simulink model "acc_with_sensor_copy"  (R2021b)
settings: Solver=FixedStepAuto  StartTime=0.0  StopTime=206  FixedStep=0.0005  RelTol=1e-3
InitFcn:
  | G=9.81;
  | m=1660;
  | rw=0.325;
  | Caf=74070;
  | Car=58525;
  | Iz=2778.5;
  | d = 1.502;
  | lf =1.1135;
  | lr =1.5065;
  | L = 2.62;
  | kph2mps=1/3.6;
values from neighbouring files (symbols this model uses):
  Leftdis_PV_switch = 2    [acc_plot_backup.m]
  s_path = [0 1.10508939428 2.2141958029 3.32141571172 4.42705301151 5.53154548532 6.63517443471 7.73808041313 8.84055018688 9.94289959674 11.0453539299 12.1480581097 ... (1001 elements, 1001x1)]    [200_100radius.mat]    (also in LV_Clothoid_S_Turn_path.mat = [0 0.966832089581 1.93621320584 2.90214024471 3.86476766313 ; NEDC_path.mat = [0 0.414605943146 0.832514087334 1.25401518562 1.68216660344; Straight_East_into_curve.mat = [0 1.65770560069 3.32192925577 4.98420060507 6.64484613518 8; acc_plot_backup.m = Station_HV_m)
  X_path = [0 1.10508939428 2.2141958029 3.32141571172 4.42705301151 5.53154548532 6.63517443471 7.73808041313 8.84055018688 9.94289959674 11.0453539299 12.1480581097 ... (1001 elements, 1001x1)]    [200_100radius.mat]    (also in LV_Clothoid_S_Turn_path.mat = [-10 -9.03316791042 -8.06378679416 -7.09785975529 -6.1352323; NEDC_path.mat = [0 0.414605943146 0.832514087334 1.25401518562 1.68216660344; Straight_East_into_curve.mat = [0 1.65770560069 3.32192925577 4.98420060507 6.64484613518 8; acc_plot_backup.m = X_HV_m)
  Y_path = [0 -1.70364610795e-18 -7.41532896709e-18 1.46822109542e-17 4.74557362791e-17 6.12980216762e-17 9.25043977736e-17 1.24088240159e-16 1.5099156923e-16 1.7058517853e-16 1.90629227614e-16 2.09673434424e-16 ... (1001 elements, 1001x1)]    [200_100radius.mat]    (also in LV_Clothoid_S_Turn_path.mat = [0 -8.46153035536e-19 5.07382551045e-18 2.07356032218e-17 3.; NEDC_path.mat = [0 -3.50680326162e-18 -2.14111304971e-18 3.38197671014e-18 3; Straight_East_into_curve.mat = [0 1.29197709199e-18 2.81882429322e-18 3.49020462564e-17 6.7; acc_plot_backup.m = Y_HV_m)
undefined symbols (not defined in the file or in its folder): C_TICK_TIME_S, Cut_in_Secenary_flg, ENUM_ACCSTATE_DISABLED, ENUM_ACCSTATE_OFF, ENUM_ACCSTATE_STANDBY, FALSE, KVDI_ACCLongPressTime_ms, KVDI_ACCMaxActSpeed_kph, KVDI_ACCSetSpdIntial_kph, KVDI_ACCSpdLargeChange_kph, KVDI_LongPressConTime_ms, ONE_FLOAT, ONE_INT, Path_selector, R, Rw, T, TRUE, UseTTC_switch, ZERO_FLOAT, ZERO_INT
libraries: simulink x15, dspstat3 x4, simulink_extras x2, Solver_SF x1
(part 1 of 8)
settings Model: Creator=power  LastModifiedBy=power
settings DataIOCC: ReturnWorkspaceOutputs=off

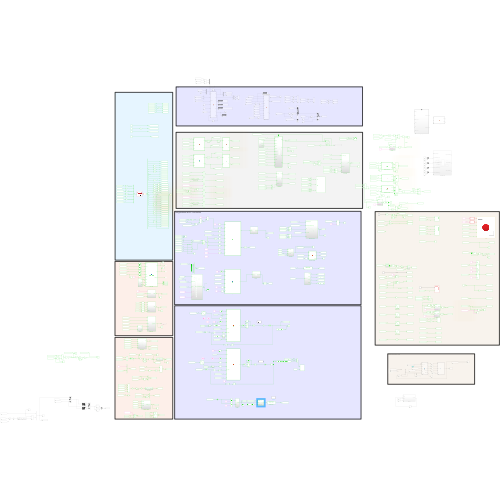
[thumbnail: Simulink's stored preview of the top-level diagram]
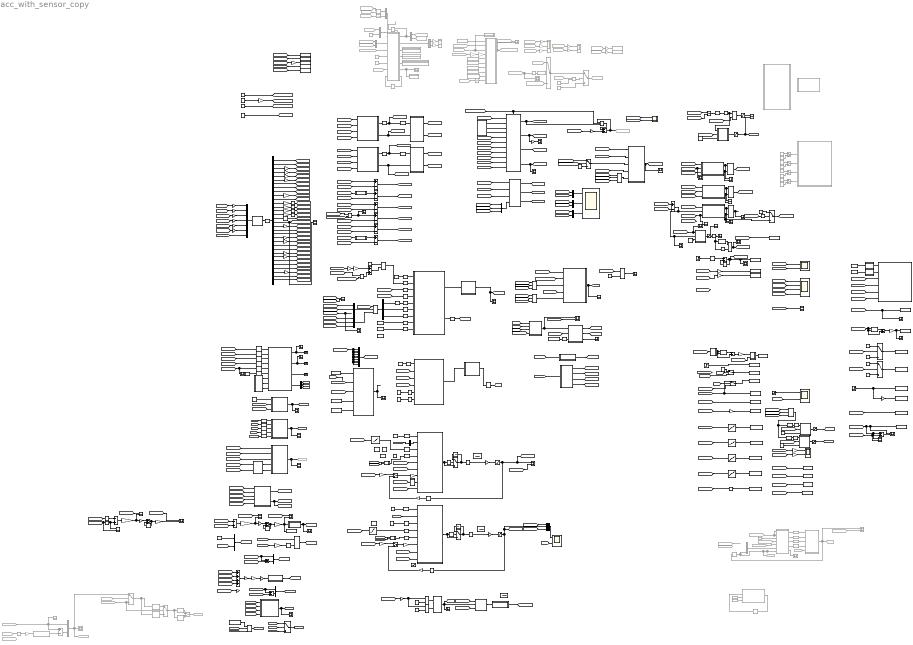
== system acc_with_sensor_copy ==
  note: Lateral MPC controller
  note: Kalman Filter
  note: Carsim
  note: Record data
  note: Longitudinal MPC controller
  note: Camera_emulator
  note: Longitudinal Constraint MPC controller
  note: Doesn't work with low speed
  note: Estimator
  note: Car_following_trajectory_planning
  1-D Lookup Table Accel Limit1 : Lookup_n-D  NumberOfTableDimensions=1  BreakpointsForDimension1=[0,5,20,30]  Table=[4,4,2,2]  InternalRulePriority=Speed  RndMeth=Simplest  InputSameDT=on
  1-D Lookup Table Deccel Limit2 : Lookup_n-D  NumberOfTableDimensions=1  BreakpointsForDimension1=[0,5,20,30]  Table=[-5,-5,-2.5,-2.5]  InternalRulePriority=Speed  RndMeth=Simplest  InputSameDT=on
  1-D Lookup Table Jerk LowLimit1 : Lookup_n-D  NumberOfTableDimensions=1  BreakpointsForDimension1=[0,5,20,30]  Table=[-5,-5,-2.5,-2.5]  InternalRulePriority=Speed  RndMeth=Simplest  InputSameDT=on
  1-D Lookup Table Jerk UpLimit1 : Lookup_n-D  NumberOfTableDimensions=1  BreakpointsForDimension1=[0,5,20,30]  Table=[5,5,2.5,2.5]  InternalRulePriority=Speed  RndMeth=Simplest  InputSameDT=on
  1-D Lookup Table1 : Lookup_n-D  NumberOfTableDimensions=1  BreakpointsForDimension1=[35 40 70 80]/3.6  Table=[0.01 0.01 0.0025 0.0025]  InternalRulePriority=Speed  RndMeth=Simplest  InputSameDT=on
  1-D Lookup Table2 : Lookup_n-D  NumberOfTableDimensions=1  BreakpointsForDimension1=[0 10 35 40]/3.6  Table=[0.25 0.25 0.025 0.025]  InternalRulePriority=Speed  RndMeth=Simplest  InputSameDT=on
  11:20 : Selector  Commented=on  InputPortWidth=20  IndexOptions=Index vector (dialog)  Indices=[11:20]  OutputSizes=1
  1:10 : Selector  Commented=on  InputPortWidth=20  IndexOptions=Index vector (dialog)  Indices=[1:10]  OutputSizes=1
  ACCSpdCalculation : Subsystem  Commented=on
  ACC_Mode_Selector : Subsystem
  Abs{,1..2,4} (4 alike) : Abs
  Abs6 : Abs  Commented=on
  Acceleration controller2 : MATLAB Function  TreatAsAtomicUnit=on
  Add{,1..3,13..14,16..17,20,32} (10 alike) : Sum  Inputs=+-
  Add Constant : Bias  Bias=-2
  Add Constant1 : Bias  Bias=2
  Add Constant2 : Bias  Bias=-2
  Add Constant4 : Bias  Bias=+2
  Add Constant5 : Bias  Bias=-2
  Add{4,9..10,60} (4 alike) : Sum  Inputs=-+
  Add{6,11,15,18,62} (5 alike) : Sum
  Add26 : Sum  Commented=on  Inputs=+-
  Add56 : Sum  Inputs=++++
  Camera_NEW : MATLAB Function  TreatAsAtomicUnit=on
  CarSim S-Function : Solver_SF/CarSim S-Function  Priority=1  SIMFILE=simfile.sim  Run_RTs=off  vs_state_ind=Run  StopMode_ind=Vehicle Model
  Compare To Constant2 : simulink/Logic and Bit Operations/Compare To Constant  Commented=on  relop=>  const=.015  OutDataTypeStr=boolean
  Compare To Constant4 : simulink/Logic and Bit Operations/Compare To Constant  relop===  const=0  OutDataTypeStr=boolean
  Compare To Constant5 : simulink/Logic and Bit Operations/Compare To Constant  relop=>=  const=2  OutDataTypeStr=boolean
  Constant : Constant  Value=0  SampleTime=0.1
  Constant10 : Constant  Value=0.1
  Constant11 : Constant  Value=45  SampleTime=0.1
  Constant111 : Constant  Value=10
  Constant{12..13,24,45} (4 alike) : Constant  Commented=on  OutDataTypeStr=boolean
  Constant14 : Constant  Value=1270+22*4+88.6+54.4  SampleTime=0.1
  Constant{15,39,46..47} (4 alike) : Constant  Commented=on  Value=0  OutDataTypeStr=boolean
  Constant{9,16,28,40,58,92} (6 alike) : Constant
  Constant17 : Constant  Value=0.3
  Constant18 : Constant  Value=0.025
  Constant19 : Constant  Value=0  SampleTime=0.1
  Constant2 : Constant  Value=2
  Constant20 : Constant  Value=10
  Constant21 : Constant  Value=10  SampleTime=0.1
  Constant{7,22,29,36,49,53} (6 alike) : Constant  Value=1.5
  Constant23 : Constant  Value=1.5  SampleTime=0.1
  Constant25 : Constant  Commented=on  Value=0.3
  Constant26 : Constant  Value=X_path
  Constant27 : Constant  Value=Y_path
  Constant3 : Constant  Value=0.1
  Constant30 : Constant  Value=35
  Constant31 : Constant  Value=3
  Constant32 : Constant  Value=30
  Constant33 : Constant  Value=5
  Constant34 : Constant  Value=-3
  Constant35 : Constant  Value=-5
  Constant37 : Constant  Commented=on  Value=0.1
  Constant38 : Constant  Commented=on  Value=0
  Constant4 : Constant  Value=0.0025
  Constant41 : Constant  Value=0.01
  Constant42 : Constant  Value=0.5
  Constant43 : Constant  Value=0.0125
  Constant44 : Constant  Commented=on  Value=100
  Constant48 : Constant  Commented=on  Value=75
  Constant5 : Constant  Value=0.2
  Constant50 : Constant  Commented=on  Value=3
  Constant52 : Constant  Commented=on  Value=1.015
  Constant54 : Constant  Commented=on  Value=2.910-1.015
  Constant55 : Constant  Commented=on  Value=1270+22*4+88.6+54.4
  Constant56 : Constant  Commented=on  Value=0.1
  Constant57 : Constant  Commented=on  Value=73922.12
  Constant59 : Constant  Commented=on  Value=54682
  Constant6 : Constant  Value=2.5
  Constant60 : Constant  Commented=on  Value=15/3.6
  Constant61 : Constant  Commented=on  Value=0
  Constant62 : Constant  Value=Leftdis_PV_switch
  Constant63 : Constant  Value=0
  Constant67 : Constant  SampleTime=0.1
  Constant8 : Constant  SampleTime=0.1
  Cos : Trigonometry  Operator=tan
  Cut-in strategy : Subsystem
  Delay{,3..4,7} (4 alike) : Delay  DelayLength=1  SampleTime=0.1
  Delay1 : Delay  DelayLength=1
  Delay10 : Delay  Commented=on  DelayLength=1  InitialConditionSource=Input port  InitialCondition=[50/3.6 0]'  SampleTime=0.1
      settings: InputPortMap=u0,p4
  Delay2 : Delay  DelayLength=1  InitialConditionSource=Input port  SampleTime=0.1
      settings: InputPortMap=u0,p4
  Delay48 : Delay  Commented=on  DelayLength=1  InitialCondition=[1 0;0 1]  SampleTime=0.1
  Delay49 : Delay  Commented=on  DelayLength=1  InitialConditionSource=Input port  InitialCondition=[50/3.6 0]'  SampleTime=0.1
      settings: InputPortMap=u0,p4
  Delay5 : Delay  Commented=on  DelayLength=1  SampleTime=0.1
  Delay50 : Delay  DelayLength=1
  Delay6 : Delay  DelayLength=1  InitialConditionSource=Input port  SampleTime=0.1
      settings: InputPortMap=u0,p4
  Delay8 : Delay  Commented=on  DelayLength=1  SampleTime=0.1
  Delay9 : Delay  DelayLength=1  InitialConditionSource=Input port  ExternalReset=Rising  SampleTime=0.1
      settings: InputPortMap=u0,r5,p4
  Demux : Demux  Outputs=32
  Demux14 : Demux
  Demux2 : Demux  Outputs=[10]
  Demux3 : Demux  Outputs=3
  Demux6 : Demux  Commented=on  Outputs=2
  Demux8 : Demux  Commented=on  Outputs=2
  Detect Increase : simulink/Logic and Bit Operations/Detect Increase  vinit=0.0  OutDataTypeStr=boolean
  Display{,4..7} (5 alike) : Display  Commented=on
      Display4 settings: Format=bank
      Display5 settings: Format=bank
      Display6 settings: Format=bank
      Display7 settings: Format=bank
  Divide : Product  Inputs=*/
  Divide1 : Product  Inputs=*/
  Estimation_TTCx_PV : MATLAB Function  TreatAsAtomicUnit=on
  Estimation_TTCx_PV1 : MATLAB Function  TreatAsAtomicUnit=on
  Estimation_TTCx_PV2 : MATLAB Function  TreatAsAtomicUnit=on
  Estimation_TTCy_PV : MATLAB Function  Commented=on  TreatAsAtomicUnit=on
  From149 : From  Commented=on  GotoTag=Ax_HV_mps2
  From157 : From  Commented=on  GotoTag=Vx_p
  From159 : From  Commented=on  GotoTag=ACCSetSpeed_mps
  From{80,160,237,247..248,253} (6 alike) : From  Commented=on  GotoTag=Vx_HV_mps
  From161 : From  Commented=on  GotoTag=Ax_HV_mps2
  From163 : From  Commented=on  GotoTag=RR
  From{166,180,232,238} (4 alike) : From  Commented=on  GotoTag=Vy_HV_mps
  From{167,219,234,258,273} (5 alike) : From  Commented=on  GotoTag=Vy_e_output
  From175 : From  Commented=on  GotoTag=Ry
  From188 : From  Commented=on  GotoTag=x_translate
  From193 : From  Commented=on  GotoTag=Ry
  From216 : From  Commented=on  GotoTag=Yaw_rate_radps
  From217 : From  Commented=on  GotoTag=Yaw_rate_radps
  From221 : From  Commented=on  GotoTag=Steer_SW_deg
  From233 : From  Commented=on  GotoTag=Ay_HV_mps2
  From239 : From  Commented=on  GotoTag=Estimated_Vx_mps
  From241 : From  Commented=on  GotoTag=Yaw_rate_radps
  From242 : From  Commented=on  GotoTag=Vy_e_Small_YawRate
  From243 : From  Commented=on  GotoTag=Ax_HV_mps2
  From244 : From  Commented=on  GotoTag=Vy_e_Small_YawRate
  From245 : From  Commented=on  GotoTag=ax_c_old
  From246 : From  Commented=on  GotoTag=Ay_HV_mps2
  From255 : From  Commented=on  GotoTag=Estimated_Vy_mps
  From257 : From  Commented=on  GotoTag=Estimated_Vy_mps
  Gain : Gain  Gain=0.25
  Gain{1,9..10,15,47..49,58} (8 alike) : Gain  Gain=1/3.6
  Gain{11,17,45,56} (4 alike) : Gain  Gain=0.1
  Gain12 : Gain  Gain=0.5
  Gain{6,8,13,19..21,31..32} (8 alike) : Gain  Gain=3.6
  Gain{14,27,30,42} (4 alike) : Gain  Gain=pi/180
  Gain18 : Gain  Gain=[0:9]
  Gain22 : Gain  Gain=0.5
  Gain23 : Gain  Gain=20
  Gain{24..26,34} (4 alike) : Gain  Gain=1/20
  Gain28 : Gain  Gain=20
  Gain3 : Gain  Gain=9.81
  Gain{33,36..38} (4 alike) : Gain
  Gain35 : Gain  Gain=-1
  Gain4 : Gain  Gain=9.81
  Gain{40,43,51..55,80..81} (9 alike) : Gain  Commented=on  Gain=3.6
  Gain41 : Gain  Commented=on  Gain=1/20
  Gain44 : Gain  Commented=on  Gain=pi/180
  Gain46 : Gain  Commented=on  Gain=0.1
  Gain5 : Gain  Gain=180/pi
  Gain50 : Gain  Gain=9.81
  Gain{57,59..61} (4 alike) : Gain  Gain=pi/30
  Gain72 : Gain  Gain=180/pi
  Goto31 : Goto  Commented=on  GotoTag=ax_c_old
  Goto44 : Goto  Commented=on  GotoTag=spd_acc
  Goto49 : Goto  Commented=on  GotoTag=Estimated_Vx_mps
  Goto58 : Goto  Commented=on  GotoTag=RR
  Goto84 : Goto  Commented=on  GotoTag=Estimated_Vy_mps
  Goto90 : Goto  Commented=on  GotoTag=Vy_e_Small_YawRate
  Goto91 : Goto  Commented=on  GotoTag=Vy_e_output
  Goto93 : Goto  Commented=on  GotoTag=LeftDis_PV_multi
  Goto95 : Goto  Commented=on  GotoTag=y_translate
  IC : InitialCondition  Value=0
  Kalman_Filter_LatSpd1 : MATLAB Function  Commented=on  TreatAsAtomicUnit=on
  Latch : Subsystem
  LateralMotionKF1 : MATLAB Function  Commented=on  TreatAsAtomicUnit=on
  Logical Operator : Logic  Operator=NOT  AllPortsSameDT=off  OutDataTypeStr=boolean
  Logical Operator3 : Logic  AllPortsSameDT=off  OutDataTypeStr=boolean
  MATLAB Function1 : MATLAB Function  TreatAsAtomicUnit=on
  MATLAB Function10 : MATLAB Function  TreatAsAtomicUnit=on
  MATLAB Function13 : MATLAB Function  TreatAsAtomicUnit=on
  MATLAB Function17 : MATLAB Function  TreatAsAtomicUnit=on
  MATLAB Function3 : MATLAB Function  TreatAsAtomicUnit=on
  MATLAB Function4 : MATLAB Function  TreatAsAtomicUnit=on
  MATLAB Function5 : MATLAB Function  TreatAsAtomicUnit=on
  MATLAB Function6 : MATLAB Function  TreatAsAtomicUnit=on
  MPC : MATLAB Function  Commented=on  TreatAsAtomicUnit=on
  MPC_ACC : MATLAB Function  TreatAsAtomicUnit=on
  MPC_Bicycle_LDC1 : MATLAB Function  TreatAsAtomicUnit=on
  Manual Switch{,1,11..12} (4 alike) : ManualSwitch  Commented=on
  Manual Switch10 : ManualSwitch  Commented=on  CurrentSetting=0
  Manual Switch5 : ManualSwitch
  Manual Switch6 : ManualSwitch
  Manual Switch9 : ManualSwitch
  Min{,1..4} (5 alike) : MinMax  Inputs=2
  Multiport Switch{,1..4} (5 alike) : MultiPortSwitch  DataPortOrder=Zero-based contiguous  Inputs=2  DiagnosticForDefault=None  zeroidx=on
  Multiport Switch5 : MultiPortSwitch  Inputs=2
  Mux : Mux  Inputs=7
  Mux1 : Mux  Inputs=2
  Mux10 : Mux  Commented=on  Inputs=2
  Mux11 : Mux  Commented=on  Inputs=2
  Mux14 : Mux  Inputs=[1 19]
  Mux15 : Mux  Commented=on  Inputs=[1 19]
  Mux16 : Mux  Inputs=[1 19]
  Mux17 : Mux  Commented=on  Inputs=2
  Mux2 : Mux  Inputs=2
  Mux20 : Mux  Inputs=[1 19]
  Mux3 : Mux  Inputs=2
  Mux{4,6..8} (4 alike) : Mux  Inputs=3
  Mux5 : Mux  Inputs=10
  Mux9 : Mux  Commented=on  Inputs=[3 1 1 1]
  PV_trajectory_planning : Subsystem
  Product : Product
  Product2 : Product
  QP_logitudinal1 : MATLAB Function  Commented=on  TreatAsAtomicUnit=on
  Quantizer{1..6} (6 alike) : Quantizer  QuantizationInterval=0.02
  R selector : Subsystem
  R selector1 : Subsystem
  R1 : Constant  Value=0.5
  Radians to Degrees1 : simulink_extras/Transformations/Radians to Degrees
  Radians to Degrees2 : simulink_extras/Transformations/Radians to Degrees
  Rate Transition{1..5,18} (6 alike) : RateTransition  OutPortSampleTime=0.1
  Relational Operator : RelationalOperator  OutDataTypeStr=boolean  RndMeth=Simplest
  Relational Operator1 : RelationalOperator  Operator=<=  OutDataTypeStr=boolean  RndMeth=Simplest
  Relational Operator2 : RelationalOperator  Operator=isNaN  OutDataTypeStr=boolean  RndMeth=Simplest
  Relational Operator3 : RelationalOperator  Commented=on  OutDataTypeStr=boolean  RndMeth=Simplest
  Relational Operator4 : RelationalOperator  Operator=isNaN  OutDataTypeStr=boolean  RndMeth=Simplest
  Reshape : Reshape  Commented=on
  Saturation : Saturate  UpperLimit=100  LowerLimit=-100
  Saturation1 : Saturate  UpperLimit=10  LowerLimit=0
  Saturation2 : Saturate  UpperLimit=30/3.6  LowerLimit=5/3.6
  Saturation3 : Saturate  UpperLimit=720  LowerLimit=-720
  Saturation4 : Saturate  UpperLimit=400  LowerLimit=-400
  Saturation5 : Saturate  UpperLimit=2.5  LowerLimit=0
  Saturation6 : Saturate  UpperLimit=2.5  LowerLimit=0
  Saturation7 : Saturate  UpperLimit=10  LowerLimit=0
  Scope{,3..4,6..10,14..15,20,24,26,31..32,34,46,49,52,56,58..59,61,63..69,76,159} (32 alike) : Scope
  Scope{1..2,5,13,16..19,22,25,27,33,42..44,70..72,75} (19 alike) : Scope  NumInputPorts=2
  Scope11 : Scope  NumInputPorts=3
  Scope12 : Scope  NumInputPorts=4
  Scope21 : Scope  Commented=on  NumInputPorts=2
  Scope{23,30,36,38,41} (5 alike) : Scope  Commented=on
  Scope50 : Scope  Commented=on  NumInputPorts=2
  Smooth Switch : Subsystem
  Smooth Switch1 : Subsystem
  Smooth_Switch1 : Subsystem  mask{tau=0.3, IC=0, T=0.1}
      mask prompts: tau "Time constant"; T "Sample time"
      mask Display:
      | fprintf('Discrete first order \n\n')
      | fprintf(['tau=' num2str(tau) '    IC=' num2str(IC)])
  Smooth_Switch2 : Subsystem  mask{tau=0.3, IC=0, T=0.1}
      mask prompts: tau "Time constant"; T "Sample time"
      mask Display:
      | fprintf('Discrete first order \n\n')
      | fprintf(['tau=' num2str(tau) '    IC=' num2str(IC)])
  Step : Step  Time=0  Before=1.5  After=1.5  SampleTime=0
  Step1 : Step  Time=0  Before=1.5  After=1.5  SampleTime=0
  Step2 : Step  Time=0  After=0.1  SampleTime=0
  Step3 : Step  Time=0  Before=5  After=5  SampleTime=0.1
  Subsystem : Subsystem
  Subsystem1 : Subsystem
  Subsystem16 : Subsystem
  Subsystem17 : Subsystem
  Subsystem2 : Subsystem
  Subsystem3 : Subsystem
  Subsystem4 : Subsystem
  Subsystem5 : Subsystem
  Subsystem6 : Subsystem  Commented=on
  Subsystem7 : Subsystem
  Subsystem8 : Subsystem
  Switch : Switch  Criteria=u2 > Threshold
  Switch{1,8,11..13} (5 alike) : Switch  Criteria=u2 ~= 0
  Switch10 : Switch  Commented=on
  Switch2 : Switch  Commented=on  Criteria=u2 ~= 0
  Switch3 : Switch  Commented=on  Criteria=u2 > Threshold
  Switch4 : Switch  Criteria=u2 > Threshold
  Switch5 : Switch  Threshold=8
  Switch6 : Switch  Threshold=8
  Switch9 : Switch  Commented=on
  T : Gain  Gain=0.1
  T1 : Gain  Gain=0.1
  Terminator1 : Terminator
  Terminator2 : Terminator
  Terminator3 : Terminator
  To Workspace : ToWorkspace  VariableName=X_HV_m  SampleTime=-1
  To Workspace1 : ToWorkspace  VariableName=Y_HV_m  SampleTime=-1
  To Workspace10 : ToWorkspace  VariableName=TH  SampleTime=-1
  To Workspace11 : ToWorkspace  VariableName=RR  SampleTime=-1
  To Workspace12 : ToWorkspace  VariableName=Desired_distance  SampleTime=-1
  To Workspace13 : ToWorkspace  VariableName=C_tick_time  SampleTime=-1
  To Workspace14 : ToWorkspace  VariableName=Ax_HV_mps2  SampleTime=-1
  To Workspace15 : ToWorkspace  VariableName=V_ref_kph  SampleTime=-1
  To Workspace16 : ToWorkspace  VariableName=Ax_Up_Limit  SampleTime=-1
  To Workspace17 : ToWorkspace  VariableName=Ax_Low_Limit  SampleTime=-1
  To Workspace18 : ToWorkspace  VariableName=Jerk_x_Up_Limit  SampleTime=-1
  To Workspace19 : ToWorkspace  VariableName=Jerk_x_Low_Limit  SampleTime=-1
  To Workspace2 : ToWorkspace  VariableName=Yaw_HV_deg  SampleTime=-1
  To Workspace20 : ToWorkspace  VariableName=Acc_Mode  SampleTime=-1
  To Workspace21 : ToWorkspace  VariableName=Ay_Low_Limit  SampleTime=-1
  To Workspace22 : ToWorkspace  VariableName=Jerk_y_Up_Limit  SampleTime=-1
  To Workspace23 : ToWorkspace  VariableName=Jerk_y_Low_Limit  SampleTime=-1
  To Workspace24 : ToWorkspace  VariableName=Ay_HV_mps2  SampleTime=-1
  To Workspace25 : ToWorkspace  VariableName=y_error  SampleTime=-1
  To Workspace26 : ToWorkspace  VariableName=Steer_SW_deg  SampleTime=-1
  To Workspace29 : ToWorkspace  VariableName=TTC  SampleTime=-1
  To Workspace3 : ToWorkspace  VariableName=Station_HV_m  SampleTime=-1
  To Workspace30 : ToWorkspace  VariableName=X_APV_m  SampleTime=0.1
  To Workspace31 : ToWorkspace  VariableName=Y_APV_m  SampleTime=0.1
  To Workspace32 : ToWorkspace  VariableName=APV_kph  SampleTime=0.1
  To Workspace34 : ToWorkspace  VariableName=Ax_APV_mps2  SampleTime=0.1
  To Workspace36 : ToWorkspace  VariableName=Station_APV_m  SampleTime=0.1
  To Workspace4 : ToWorkspace  VariableName=Jerk_y  SampleTime=-1
  To Workspace40 : ToWorkspace  VariableName=Yaw_Est_deg  SampleTime=-1
  To Workspace42 : ToWorkspace  Commented=on  VariableName=Vy_HV_kph  SampleTime=-1
  To Workspace43 : ToWorkspace  Commented=on  VariableName=Vy_e_output  SampleTime=-1
  To Workspace5 : ToWorkspace  VariableName=Ay_Up_Limit  SampleTime=-1
  To Workspace6 : ToWorkspace  VariableName=HV_kph  SampleTime=-1
  To Workspace7 : ToWorkspace  VariableName=PV_kph  SampleTime=-1
  To Workspace8 : ToWorkspace  VariableName=Jerk_x  SampleTime=-1
  To Workspace9 : ToWorkspace  VariableName=TH_ref  SampleTime=0.1
  Transfer Fcn2 : TransferFcn  Denominator=[0.3 1]
  Transfer Fcn3 : TransferFcn  Denominator=[0.3 1]
  Transfer Fcn4 : TransferFcn  Denominator=[0.3 1]
  Unit Delay : UnitDelay  SampleTime=-1  HasFrameUpgradeWarning=on
  Unit Delay2 : UnitDelay  SampleTime=-1  HasFrameUpgradeWarning=on
  Unit Delay4 : UnitDelay  Commented=on  SampleTime=0.1  HasFrameUpgradeWarning=on
  Unit Delay5 : UnitDelay  Commented=on  SampleTime=0.1  HasFrameUpgradeWarning=on
  V_rel Estimation : Subsystem
  Vx4 : Scope  Commented=on  NumInputPorts=3
  Vx5 : Scope  Commented=on  NumInputPorts=2
  Vx6 : Scope  Commented=on  NumInputPorts=2
  XY Graph : Record  FileSettingsInternal="{\"entries\":[{\"content\":{\"excelSettings\":{\"content\":{},\"type\":\"Streamout.ExcelSettings\"}},\"type\":\"Streamout.FileSettingStorage\",\"uuid\":\"ae1c5602-517a-41a1-a61f-ee7d5eb1a325\"}],\"packageUris\":[\"http://schema.mathworks.com/mf0/streamout_blocks/R2020a\"],\"version\":\"1.0\"}"  Layout=[1 1]  SignalsInternal="{\"entries\":[{\"content\":{\"signals\":[{\"content\":{\"blockPath\":[\"acc_with_sensor/XY Graph\"],\"channel\":[],\"dimensions\":[1],\"domain\":\"acc_with_sensor/XY Graph\",\"lineColor\":\"#a2142f\",\"plots\":[1],\"port\":1,\"sid\":[\"\"],\"signalID\":8457,\"signalName\":\"x\"},\"type\":\"RecordBlkView.Signal\",\"uuid\":\"a7bf0323-9e6d-485d-a474-0a9d372fb7b1\"},{\"content\":{\"blockPath\":[\"acc_with_sensor/XY Graph\"],\"channel\":[],\"dimensions\":[1],\"domain\":\"acc_with_sensor/XY Graph\",\"lineColor\":\"#139fff\",\"plots\":[1],\"port\":2,\"sid\":[\"\"],\"signalID\":8461,\"signalName\":\"y\"},\"type\":\"RecordBlkView.Signal\",\"uuid\":\"749632c3-9221-4843-a7a6-8451e6d0203a\"},{\"content\":{\"blockPath\":[\"acc_with_sensor/XY Graph\"],\"channel\":[],\"dimensions\":[1],\"domain\":\"acc_with_sensor/XY Graph\",\"lineColor\":\"#64d413\",\"plots\":[1],\"port\":3,\"sid\":[\"\"],\"signalID\":8465,\"signalName\":\"X_HV\"},\"type\":\"RecordBlkView.Signal\",\"uuid\":\"02048bb8-c637-427d-932f-1a61c452e62e\"},{\"content\":{\"blockPath\":[\"acc_with_sensor/XY Graph\"],\"channel\":[],\"dimensions\":[1],\"domain\":\"acc_with_sensor/XY Graph\",\"lineColor\":\"#ff13a6\",\"plots\":[1],\"port\":4,\"sid\":[\"\"],\"signalID\":8469,\"signalName\":\"Y_HV\"},\"type\":\"RecordBlkView.Signal\",\"uuid\":\"63ffdeac-a074-4ec1-8896-dcf10e1ec4b5\"},{\"content\":{\"blockPath\":[\"acc_with_sensor/XY Graph\"],\"channel\":[],\"dimensions\":[1],\"domain\":\"acc_with_sensor/XY Graph\",\"lineColor\":\"#ff6929\",\"plots\":[1],\"port\":5,\"sid\":[\"\"],\"signalID\":8473,\"signalName\":\"X_PV\"},\"type\":\"RecordBlkView.Signal\",\"uuid\":\"92c1fdf2-3407-44d2-b4da-fad837cd08fa\"},{\"content\":{\"blockPath\":[\"acc_with_sensor/XY Graph\"],\"channel\":[],\"dimensions\":[1],\"domain\":\"acc_with_sensor/XY Graph\",\"lineColor\":\"#b746ff\",\"plots\":[1],\"port\":6,\"sid\":[\"\"],\"signalID\":8477,\"signalName\":\"Y_PV\"},\"type\":\"RecordBlkView.Signal\",\"uuid\":\"c8381700-cb77-42bf-bc65-a1a6c0c1696f\"}]},\"type\":\"RecordBlkView.InputSignals\",\"uuid\":\"40a95d25-711b-4f06-a3ff-602c17e43ef4\"}],\"packageUris\":[\"http://schema.mathworks.com/mf0/streamout_blocks/R2020a\"],\"version\":\"1.0\"}"  VisualizationBindings="{\"xyplotplugin\":{\"info\":[{\"series\":[{\"bindingParametersList\":[{\"parameter\":\"X-Axis\",\"signalID\":8465,\"signalName\":\"X_HV\"},{\"parameter\":\"Y-Axis\",\"signalID\":8469,\"signalName\":\"Y_HV\"}],\"seriesID\":54143},{\"bindingParametersList\":[{\"parameter\":\"X-Axis\",\"signalID\":8473,\"signalName\":\"X_PV\"},{\"parameter\":\"Y-Axis\",\"signalID\":8477,\"signalName\":\"Y_PV\"}],\"seriesID\":48964},{\"bindingParametersList\":[{\"parameter\":\"X-Axis\",\"signalID\":8457,\"signalName\":\"x\"},{\"parameter\":\"Y-Axis\",\"signalID\":8461,\"signalName\":\"y\"}],\"seriesID\":3520}],\"subplotID\":1}]}}"  CompatibilityTag=XY
  Zero-Order Hold{1..4,6,8..14,17..25,132..136} (26 alike) : ZeroOrderHold  SampleTime=0.1
  Zero-Order Hold{26..27,29,36} (4 alike) : ZeroOrderHold  Commented=on  SampleTime=0.1
  acceleration_apr1 : Subsystem
  acceleration_apr4 : Subsystem
  ascending : dspstat3/Sort  Commented=on  otype=Value  dir=Ascending  sortAlg=Quick sort  roundingMode=Floor  overflowMode=off  accumDataTypeStr=Inherit: Same as product output  accumLastDataTypeStr=Inherit: Same as product output
      settings: SourceProductBaseCode=DS
  car_length : Bias  Bias=-4.5
  car_length1 : Bias  Bias=4.5
  car_length2 : Bias  Bias=-4.5
  car_length3 : Bias  Bias=4.5
  cmd_limiter1 : Subsystem
  cmd_limiter4 : Subsystem
  descending : dspstat3/Sort  Commented=on  otype=Value  dir=Descending  sortAlg=Quick sort  roundingMode=Floor  overflowMode=off  accumDataTypeStr=Inherit: Same as product output  accumLastDataTypeStr=Inherit: Same as product output
      settings: SourceProductBaseCode=DS
  dist_safe : Bias  Bias=-2
  divide : Subsystem
  divide1 : Subsystem
  divide2 : Subsystem
  divide3 : Subsystem
  global to local2 : Subsystem
  global to local3 : Subsystem
  preview : Subsystem
  r/l : Gain  Gain=0.33415/1.675
  r/l1 : Gain  Gain=0.33415/1.675
  record_delta_x : Subsystem
  record_delta_yaw : Subsystem
  relative_dynamic_estimated : Subsystem  Commented=on
  rolling radius : Gain  Gain=0.325
  rolling_avg : Subsystem  Commented=on
  sample time1 : Gain  Gain=1/0.1
  sample time2 : Gain  Gain=1/0.1
  way2 : Goto  Commented=on  GotoTag=LeftDis_Camera
  tag scope: RAx_APV=global, RAx_PV=global, RR_APV=global, RR_PV=global, RVx_APV=global, RVx_PV=global, Vx_HV_mps=global
  wires:
  Demux/1 -> [X_HV_m]
  CarSim S-Function/1 -> Zero-Order Hold18/1
  Demux/2 -> [Y_HV_m]
  Demux/3 -> Gain9/1
  Demux/4 -> Gain10/1
  Demux/5 -> Gain3/1
  Demux/6 -> Gain4/1
  [Vx_PV_mps] -> Add1/1
  [Vx_HV_mps] -> Add1/2
  acceleration_apr4/1(acc_a) -> Add2/1  "PV"
  [Ax_HV_mps2] -> Add2/2  "HV"
  Constant14/1 -> Zero-Order Hold17/1
  Subsystem2/4(Pb_RR) -> [Braking_Pressure_RR]
  Product/1 -> Zero-Order Hold6/1
  [Driving_Brk_Cmd] -> Subsystem2/1(T_cmd)
  Subsystem2/1(Pb_LF) -> [Braking_Pressure_LF]
  Acceleration controller2/2(Tb) -> [Driving_Brk_Cmd]
  Acceleration controller2/3(Rtotal) -> Scope159/1
  Subsystem2/3(Pb_RL) -> [Braking_Pressure_RL]
  [Ax_HV_mps2] -> Zero-Order Hold9/1
  [Vx_HV_mps] -> Zero-Order Hold8/1
  Acceleration controller2/1(Tr) -> [Driving_Torque_Cmd]  "Torque"
  Subsystem2/2(Pb_RF) -> [Braking_Pressure_RF]
  Gain9/1 -> [Vx_HV_mps]
  Gain10/1 -> [Vy_HV_mps]
  Gain3/1 -> [Ax_HV_mps2]
  Gain4/1 -> [Ay_HV_mps2]
  Gain22/1 -> Mux/1  "Driving_Torque_FL"
  Gain12/1 -> Mux/2  "Driving_Torque_FR"
  Zero-Order Hold6/1 -> MATLAB Function1/2(Yref)
  Zero-Order Hold8/1 -> MATLAB Function1/3(Vx)
  Zero-Order Hold9/1 -> MATLAB Function1/4(ax)
  Zero-Order Hold10/1 -> MATLAB Function1/5(D_rel)
  Zero-Order Hold11/1 -> MATLAB Function1/6(V_rel)
  Zero-Order Hold12/1 -> MATLAB Function1/7(ax_rel)
  Zero-Order Hold13/1 -> MATLAB Function1/8(Qs)
  Zero-Order Hold14/1 -> MATLAB Function1/9(Rs)
  Abs/1 -> divide/1(dividend)
  Mux1/1 -> Scope11/1  "RR"
  [RR] -> Mux1/1  "RR"
  [RR_est] -> Mux1/2  "Est"
  [RVx] -> Mux2/1  "RV"
  [RV_est] -> Mux2/2  "Est"
  [RAx] -> Mux3/1  "RA"
  [RA_est] -> Mux3/2  "Est"
  Mux2/1 -> Scope11/2  "RV"
  Mux3/1 -> Scope11/3  "RA"
  [Braking_Pressure_RF] -> Gain36/1
  Gain33/1 -> Mux/3  "Driving_Torque_LF"
  [Braking_Pressure_LF] -> Gain33/1
  [Braking_Pressure_RL] -> Gain37/1
  Gain36/1 -> Mux/4  "Driving_Torque_RF"
  Gain38/1 -> Mux/6  "Driving_Torque_RR"
  Gain37/1 -> Mux/5  "Driving_Torque_RL"
  [Braking_Pressure_RR] -> Gain38/1
  [Braking_Pressure_LF] -> Scope12/1  "LF"
  [Braking_Pressure_RF] -> Scope12/2  "RF"
  [Braking_Pressure_RL] -> Scope12/3  "RL"
  [Braking_Pressure_RR] -> Scope12/4  "RR"
  MATLAB Function1/2(Y) -> Add Constant1/1  "MPC"
  Gain8/1 -> Scope18/1  "HV"
  Gain13/1 -> Scope18/2  "PV"
  [Vx_HV_mps] -> Acceleration controller2/2(Vxh)
  Zero-Order Hold17/1 -> Acceleration controller2/3(m)
  Zero-Order Hold18/1 -> Demux/1
  [RR] -> Scope13/2  "RR"
  Step/1 -> Scope2/1  "TH_limit"
  [TH] -> Scope2/2  "TH"
  Demux3/3 -> Zero-Order Hold12/1
  Zero-Order Hold3/1 -> MATLAB Function1/1(mode)
  [Driving_Torque] -> Gain22/1
  [Driving_Torque] -> Gain12/1
  [Ax_HV_mps2] -> Scope17/2  "ax_out"
  [Vx_HV_mps] -> Gain8/1  "HV"
  [Vx_PV_mps] -> Gain13/1  "PV"
  Demux3/2 -> Zero-Order Hold11/1
  [Driving_Torque_Cmd] -> Smooth_Switch2/1(In1)
  [Vx_HV_mps] -> MPC_ACC/3(Vx)
  [Ax_HV_mps2] -> MPC_ACC/4(ax)
  Constant92/1 -> Zero-Order Hold1/1
  Constant5/1 -> Zero-Order Hold2/1
  Constant2/1 -> Subsystem/4(Ax_max)
  Constant6/1 -> Subsystem/5(Jx_max)
  [Vx_HV_mps] -> Subsystem/3(VehSpd)
  [Vx_p] -> MPC_ACC/2(vx_p)
  Subsystem/1("VREF_LongiVehSpdRef_mps ") -> Scope4/1  "mps"
  Zero-Order Hold1/1 -> MPC_ACC/5(Qs)
  Zero-Order Hold2/1 -> MPC_ACC/6(Rs)
  MATLAB Function1/1(u) -> cmd_limiter1/1(ax_cmd)  "cmd"
  Add2/1 -> [RAx_PV]
  Add1/1 -> [RVx_PV]
  [Acc_Mode] -> ?
  [ACCSetSpeed_mps] -> Mux5/10, Mux5/9, Mux5/8, Mux5/7, Mux5/6, Mux5/5, Mux5/4, Mux5/3, Mux5/2, Mux5/1
  Add Constant/1 -> Abs/1
  Constant11/1 -> Gain15/1
  Gain15/1 -> [ACCSetSpeed_mps]
  Demux3/1 -> dist_safe/1
  [ACCSetSpeed_mps] -> ACC_Mode_Selector/1(ACCSetSpeed_mps)
  [VACCTargetVehAssigned_flg] -> ACC_Mode_Selector/2(VACCTargetVehNotAssigned_flg)
  [Vx_HV_mps] -> ACC_Mode_Selector/4(Vx_HV_mps)
  [Ax_HV_mps2] -> Gain17/1
  Gain17/1 -> Gain18/1
  Gain18/1 -> Add6/1
  Add6/1 -> Product/2  "Vp"
  Add Constant1/1 -> [Desired_distance]
  [Ax_PV_mps2] -> acceleration_apr4/1(acc_b)  "PV"
  Smooth_Switch2/1(Out1) -> [Driving_Torque]
  [Vx_HV_mps] -> Gain20/1  "HV"
  Gain19/1 -> To Workspace7/1  "PV"
  Gain20/1 -> To Workspace6/1  "HV"
  Subsystem4/1(new_ave) -> Delay2/1, Delay2/2, Add10/2
  Add10/1 -> sample time1/1
  Delay2/1 -> Add10/1
  sample time1/1 -> Subsystem3/1(Jerk)  "Jerk"
  Step1/1 -> To Workspace9/1  "TH_limit"
  [Desired_distance] -> Scope13/1  "Desired_distance"
  [Desired_distance] -> Switch8/1, To Workspace12/1  "Desired_distance"
  Step2/1 -> Delay3/1
  Add11/1 -> Scope31/1, To Workspace13/1, [C_tick_time], Delay/1
  Delay/1 -> Add11/2
  Delay3/1 -> Add11/1
  [Ax_HV_mps2] -> To Workspace14/1
  [ACCSetSpeed_mps] -> Subsystem/2(VehSpd_Ref)
  [ACCSetSpeed_mps] -> Gain21/1
  Gain21/1 -> To Workspace15/1
  Mux5/1 -> [Vx_p]
  Constant30/1 -> Relational Operator/2
  Relational Operator1/1 -> Latch/2(reset)
  Constant32/1 -> Relational Operator1/2
  Relational Operator/1 -> Latch/1(set)
  Gain31/1 -> Relational Operator/1, Relational Operator1/1  "kph"
  [RR_PV] -> Estimation_TTCx_PV/1(R)
  [RVx_PV] -> Estimation_TTCx_PV/2(V)
  [RAx_PV] -> Estimation_TTCx_PV/3(A)
  [Vx_HV_mps] -> 1-D Lookup Table Deccel Limit2/1
  1-D Lookup Table Deccel Limit2/1 -> To Workspace17/1
  [Vx_HV_mps] -> 1-D Lookup Table Accel Limit1/1
  1-D Lookup Table Accel Limit1/1 -> To Workspace16/1
  [Vx_HV_mps] -> 1-D Lookup Table Jerk UpLimit1/1
  [Vx_HV_mps] -> 1-D Lookup Table Jerk LowLimit1/1
  1-D Lookup Table Jerk UpLimit1/1 -> To Workspace18/1
  1-D Lookup Table Jerk LowLimit1/1 -> To Workspace19/1
  dist_safe/1 -> Zero-Order Hold10/1  "Drel"
  [Acc_Mode] -> Logical Operator/1
  Constant29/1 -> divide/3(default_value)
  divide/1(quotient) -> Saturation1/1
  Saturation1/1 -> [TH]  "TH_default"
  [X_PV_m] -> MATLAB Function3/1(Xf)
  [Y_PV_m] -> MATLAB Function3/2(Yf)
  [X_HV_m] -> MATLAB Function3/3(Xh)
  [Y_HV_m] -> MATLAB Function3/4(Yh)
  MATLAB Function3/1(RR) -> car_length/1  "RR_XY"
  Demux/7 -> [Station_HV_m]  "Station_HV"
  Constant9/1 -> Zero-Order Hold13/1
  Constant10/1 -> Zero-Order Hold14/1
  [RA_est] -> Mux6/3
  [RV_est] -> Mux6/2
  [RR_est] -> Mux6/1
  Multiport Switch2/1 -> Demux3/1
  Mux6/1 -> Multiport Switch2/3
  Multiport Switch/1 -> Add Constant5/1, Add Constant/1
  Zero-Order Hold4/1 -> MPC_ACC/1(trig)
  Multiport Switch3/1 -> ACC_Mode_Selector/3(RR)
  [Acc_Mode] -> Scope6/1
  Smooth Switch/1(ax_cmd) -> Acceleration controller2/1(axc), Scope17/1
  Multiport Switch4/1 -> ACC_Mode_Selector/5(RV)
  [Vx_HV_mps] -> divide/2(divisor)
  car_length/1 -> car_length1/1, [RR_PV]  "RR"
  Demux/8 -> [Steer_SW_deg]
  Rate Transition1/1 -> Camera_NEW/4(Yo)
  Demux14/3 -> [C2]
  Rate Transition3/1 -> Camera_NEW/2(phi_deg)
  [PrediDis] -> Zero-Order Hold136/1
  [Y_HV_m] -> Rate Transition1/1
  [X_HV_m] -> Rate Transition2/1
  [Yaw_HV_deg] -> Rate Transition3/1  "deg"
  [Station_HV_m] -> Scope14/1, Rate Transition18/1
  Rate Transition2/1 -> Camera_NEW/3(Xo)
  Rate Transition18/1 -> Camera_NEW/5(station)
  Zero-Order Hold134/1 -> Subsystem16/3("C2 ")
  [C2] -> Zero-Order Hold134/1
  [C3] -> Zero-Order Hold135/1
  Camera_NEW/3(Heading_ref) -> Terminator2/1
  [C0] -> Zero-Order Hold132/1
  Rate Transition4/1 -> Camera_NEW/1(ux_mps)
  Demux14/1 -> [C0]
  Zero-Order Hold133/1 -> Subsystem16/2(C1)
  Zero-Order Hold135/1 -> Subsystem16/4(C3)
  Subsystem17/1(PrediDis) -> Scope15/1, [PrediDis]
  Zero-Order Hold136/1 -> Subsystem16/5(PrediDis)
  [Vx_HV_mps] -> Rate Transition4/1  "mps"
  Subsystem16/1(LeftDis) -> [LeftDis_Camera], Scope3/1
  [C1] -> Zero-Order Hold133/1
  Camera_NEW/1(x_ref) -> Scope46/1, Terminator1/1
  Constant111/1 -> Subsystem17/1(Np)
  Camera_NEW/4(C) -> Demux14/1
  Demux14/2 -> [C1]
  Demux14/4 -> [C3]
  Zero-Order Hold132/1 -> Subsystem16/1(C0)
  Demux/9 -> [Yaw_HV_deg]
  [X_HV_m] -> To Workspace/1
  [Y_HV_m] -> To Workspace1/1
  [Yaw_HV_deg] -> To Workspace2/1
  [Station_HV_m] -> To Workspace3/1
  Rate Transition5/1 -> Camera_NEW/6(Ts_MPC)
  Constant3/1 -> Rate Transition5/1
  Zero-Order Hold19/1 -> MATLAB Function17/1(trig)
  Constant16/1 -> Zero-Order Hold19/1
  [y_ref] -> MATLAB Function17/2(Yref)
  Zero-Order Hold20/1 -> MATLAB Function17/3(tau)
  Constant17/1 -> Zero-Order Hold20/1
  Zero-Order Hold22/1 -> MATLAB Function17/5(Rs)
  Zero-Order Hold21/1 -> MATLAB Function17/4(Qs)
  R selector/1(Out1) -> Zero-Order Hold22/1
  1-D Lookup Table2/1 -> Zero-Order Hold21/1
  Gain14/1 -> MATLAB Function17/6(steer_angle)
  Switch/1 -> Radians to Degrees1/1, Unit Delay/1
  Saturation3/1 -> Mux8/2, [Steer_Kinematic_deg], Delay4/1  "Kinematic"
  [Steer_SW_deg] -> Mux8/3  "carsim"
  Gain23/1 -> Saturation3/1  "deg"
  Delay4/1 -> Gain24/1
  Gain24/1 -> Manual Switch5/2  "deg"
  [Ax_HV_mps2] -> MATLAB Function17/8(Ax)
  [X_HV_m] -> global to local3/1(Xc)
  [Yaw_HV_deg] -> global to local3/3(Yaw)  "deg"
  [Y_HV_m] -> global to local3/2(Yc)
  [Steer_IN_deg] -> Mux/7
  MATLAB Function17/1(u) -> Relational Operator2/1, Switch/3
  Unit Delay/1 -> Switch/1
  Relational Operator2/1 -> Switch/2
  Demux/10 -> Gain30/1
  Gain30/1 -> [Yaw_rate_radps]
  Constant26/1 -> MATLAB Function13/1(u)
  MATLAB Function13/1(y) -> XY Graph/1  "x"
  Constant27/1 -> MATLAB Function5/1(u)
  MATLAB Function5/1(y) -> XY Graph/2  "y"
  [X_HV_m] -> XY Graph/3  "X_HV"
  [Y_HV_m] -> XY Graph/4  "Y_HV"
  [Vx_HV_mps] -> Gain31/1
  [Steer_SW_deg] -> Gain34/1  "carsim"
  Gain34/1 -> Manual Switch5/1  "deg"
  Manual Switch5/1 -> Gain14/1
  Latch/1(latched) -> Scope/1, Smooth Switch1/2(Mode), [LFC_Mode]
  [Ay_HV_mps2] -> To Workspace24/1, Scope9/1
  sample time2/1 -> To Workspace4/1, Scope10/1  "Jerk"
  Delay6/1 -> Add4/1
  Add4/1 -> sample time2/1
  [Ay_HV_mps2] -> Add4/2, Delay6/2, Delay6/1
  [Vx_HV_mps] -> Switch5/2
  Switch5/1 -> To Workspace5/1
  Constant31/1 -> Switch5/1
  Constant33/1 -> Switch5/3
  Constant35/1 -> Switch6/3
  Constant34/1 -> Switch6/1
  Switch6/1 -> To Workspace21/1
  [Vx_HV_mps] -> Switch6/2
  Step3/1 -> Gain35/1, To Workspace22/1  "TH_limit"
  Gain35/1 -> To Workspace23/1
  rolling_avg/1(new_ave) -> Delay5/1
  [Steer_SW_deg] -> To Workspace26/1  "carsim"
  Constant36/1 -> Product/1
  ACC_Mode_Selector/1(Out1) -> Scope52/1, [Acc_Mode]
  Delay5/1 -> rolling_avg/2(old_ave)
  Constant37/1 -> rolling_avg/3(delta_t)  "T"
  Constant25/1 -> rolling_avg/4(tc)
  Smooth Switch1/1(ax_cmd) -> Smooth_Switch1/1(In1)
  Demux/11 -> [y_error_m]
  [y_error_m] -> Scope42/1, Add/1, Scope19/1, To Workspace25/1  "HV"
  [y_error_LV] -> Scope42/2, Add/2
  Add/1 -> Scope19/2  "add_PV"
  Subsystem1/1(Out1) -> MPC_Bicycle_LDC1/8(Vx)
  Gain26/1 -> Manual Switch9/1  "deg"
  Manual Switch9/1 -> Gain27/1
  [Steer_SW_deg] -> Gain26/1  "carsim"
  Relational Operator4/1 -> Switch4/2
  Unit Delay2/1 -> Switch4/1
  MPC_Bicycle_LDC1/1(u) -> Switch4/3, Relational Operator4/1
  Gain25/1 -> Manual Switch9/2  "deg"
  Switch4/1 -> Unit Delay2/1, Radians to Degrees2/1
  Saturation4/1 -> [Steer_Dynamic_deg], Scope25/1, Delay7/1  "mpc"
  Delay7/1 -> Gain25/1
  [Ax_HV_mps2] -> MPC_Bicycle_LDC1/9(Ax)
  [Vx_HV_mps] -> Subsystem1/1(In1)
  Gain27/1 -> MPC_Bicycle_LDC1/7(steer_angel)
  Gain28/1 -> Saturation4/1  "deg"
  [Yaw_rate_radps] -> MPC_Bicycle_LDC1/6(yaw_rate)
  [Vy_HV_mps] -> MPC_Bicycle_LDC1/5(Vy)
  Zero-Order Hold24/1 -> MPC_Bicycle_LDC1/4(Rs)
  Zero-Order Hold23/1 -> MPC_Bicycle_LDC1/3(Qs)
  R selector1/1(Out1) -> Zero-Order Hold24/1
  1-D Lookup Table1/1 -> Zero-Order Hold23/1
  [y_ref] -> Demux2/1
  Zero-Order Hold25/1 -> MPC_Bicycle_LDC1/1(trig)
  Constant40/1 -> Zero-Order Hold25/1
  [Steer_SW_deg] -> Scope25/2  "carsim"
  Constant46/1 -> Manual Switch12/1
  Constant45/1 -> Manual Switch12/2
  Manual Switch12/1 -> ACCSpdCalculation/5(VDINR_ACCSpdResInc_flg)
  Manual Switch11/1 -> ACCSpdCalculation/4(VDINR_ACCSpdSetDec_flg)
  Constant24/1 -> Manual Switch11/2
  Constant39/1 -> Manual Switch11/1
  Manual Switch10/1 -> ACCSpdCalculation/3(NVDI_ACCSystemStatePrev_enum)
  Constant15/1 -> Manual Switch10/1
  Constant13/1 -> Manual Switch10/2
  Manual Switch/1 -> ACCSpdCalculation/2(NVDI_ACCActingPrev_flg)
  Constant12/1 -> Manual Switch/2
  Constant47/1 -> Manual Switch/1
  Camera_NEW/2(y_ref) -> Scope26/1, Terminator3/1  "yref"
  MATLAB Function3/2(RD) -> [RD_PV], MATLAB Function10/2(RD)
  MATLAB Function10/1(RX) -> [RX_PV]
  MATLAB Function10/2(RY) -> [RY_PV]
  car_length1/1 -> MATLAB Function10/1(RR)  "RR"
  Switch1/1 -> [y_ref]
  [LeftDis_Camera] -> Switch1/1
  [LeftDis_PV] -> Switch1/3
  [LaneAvail_flg] -> Switch1/2  "LaneAvail_flg"
  [X_PV_m] -> XY Graph/5  "X_PV"
  [Y_PV_m] -> XY Graph/6  "Y_PV"
  [Steer_Dynamic_deg] -> Mux8/1  "Dynamic"
  Mux8/1 -> Scope1/1
  [Vx_HV_mps] -> Subsystem17/2(VehSpd_mps)
  cmd_limiter4/1(ax_cmd1) -> IC/1
  From163/1 -> ?
  Zero-Order Hold27/1 -> QP_logitudinal1/3(A_cons)
  MPC/3(M_act) -> Zero-Order Hold27/1
  Delay8/1 -> Mux9/4, MPC/7(ax_c_old), Goto31/1
  Zero-Order Hold26/1 -> QP_logitudinal1/2(f)
  MPC/4(gamma_act) -> Zero-Order Hold29/1
  From160/1 -> MPC/4(vxh)
  MPC/1(HH) -> Zero-Order Hold36/1
  From159/1 -> MPC/1(vx_p), MPC/2(vx_acc_set)
  Zero-Order Hold29/1 -> QP_logitudinal1/4(b)
  MPC/5(fesible_flag) -> Scope38/1
  Mux9/1 -> MPC/6(X_thk)
  Constant50/1 -> MPC/3(mode)
  MPC/2(ff) -> Zero-Order Hold26/1
  From245/1 -> QP_logitudinal1/5(u_old)
  Zero-Order Hold36/1 -> QP_logitudinal1/1(H)
  QP_logitudinal1/1(u) -> Scope21/1, Goto44/1, Delay8/1
  From149/1 -> Scope21/2  "ax_out"
  From161/1 -> MPC/5(axh)
  [spd_acc] -> Smooth Switch/1(Spd_acc_cmd)  "cmd"
  [Acc_Mode] -> Smooth Switch/2(Mode)
  [th_acc] -> Smooth Switch/3(TH_acc_cmd)  "cmd"
  MPC_ACC/1(u) -> cmd_limiter4/1(ax_cmd)  "cmd"
  [Steer_Dynamic_deg] -> Smooth Switch1/1(Dynamic_cmd)
  [Steer_Kinematic_deg] -> Smooth Switch1/3(Kinematic_cmd)
  [Vx_HV_mps] -> Subsystem3/2(Vx)
  Subsystem3/1(Out1) -> To Workspace8/1
  [TTC] -> Smooth Switch/4(TTC)
  [LFC_Mode] -> Scope1/2
  [Vx_HV_mps] -> 1-D Lookup Table1/1
  Radians to Degrees2/1 -> Gain28/1
  Radians to Degrees1/1 -> Gain23/1
  Demux2/1 -> MPC_Bicycle_LDC1/2(Yref)
  [Ax_HV_mps2] -> Subsystem17/3(In3)
  global to local3/1(y_path_ref10) -> way2/1, Scope24/1
  [Vx_HV_mps] -> 1-D Lookup Table2/1
  [Vx_HV_mps] -> MATLAB Function17/7(Vx)
  Smooth_Switch1/1(Out1) -> [Steer_IN_deg]
  Logical Operator/1 -> To Workspace20/1
  [Ax_HV_mps2] -> Subsystem4/1(new_value)
  [Vy_PV_mps] -> Add13/1
  [Vy_HV_mps] -> Add13/2
  Add13/1 -> [RVy_PV]
  car_length3/1 -> MATLAB Function4/1(RR)  "RR"
  MATLAB Function4/2(RY) -> [RY_APV]
  MATLAB Function4/1(RX) -> [RX_APV]
  car_length2/1 -> car_length3/1, [RR_APV]  "RR"
  MATLAB Function6/1(RR) -> car_length2/1  "RR_XY"
  [Y_HV_m] -> MATLAB Function6/4(Yh)
  [X_HV_m] -> MATLAB Function6/3(Xh)
  [Y_APV_m] -> MATLAB Function6/2(Yf)
  [X_APV_m] -> MATLAB Function6/1(Xf)
  Add14/1 -> [RVx_APV]
  [Vx_HV_mps] -> Add14/2
  Min4/1 -> Scope63/1, Add14/1
  Add16/1 -> [RVy_APV]
  [Vy_HV_mps] -> Add16/2
  [Vy_APV_mps] -> Add16/1
  MATLAB Function6/2(RD) -> MATLAB Function4/2(RD), [RD_APV]
  [RAx_APV] -> Estimation_TTCx_PV1/3(A)
  [RVx_APV] -> Scope64/1, Estimation_TTCx_PV1/2(V)
  [RR_APV] -> Estimation_TTCx_PV1/1(R)
  [Ax_APV_mps2] -> acceleration_apr1/1(acc_b)  "PV"
  Add17/1 -> [RAx_APV]
  [Ax_HV_mps2] -> Add17/2  "HV"
  acceleration_apr1/1(acc_a) -> Add17/1  "PV"
  Saturation5/1 -> Scope44/1  "TH"
  [Vx_HV_mps] -> divide1/2(divisor)
  divide1/1(quotient) -> Saturation6/1
  Add Constant2/1 -> Abs1/1
  [RR_APV] -> Manual Switch6/1
  Divide1/1 -> Saturation5/1  "TH_cal"
  Constant53/1 -> divide1/3(default_value)
  Manual Switch6/1 -> Add Constant2/1
  Saturation6/1 -> [TH_APV], Scope44/2  "TH_default"
  [RR_est] -> Manual Switch6/2
  [Vx_HV_mps] -> Divide1/2
  Abs1/1 -> divide1/1(dividend), Divide1/1
  Mux7/1 -> Multiport Switch2/2
  [RR] -> Switch8/3  "RR"
  Estimation_TTCx_PV2/2(TTC2) -> Switch13/3, Scope22/2, Min/2
  Estimation_TTCx_PV2/1(TTC1) -> Scope22/1, Min/1
  [RAx] -> Scope67/1, Estimation_TTCx_PV2/3(A)
  Switch11/1 -> To Workspace10/1  "TH"
  [X_APV_m] -> To Workspace30/1
  [Station_APV_m] -> To Workspace36/1
  [Ax_APV_mps2] -> To Workspace34/1
  [Vx_APV_mps] -> Gain32/1
  [Y_APV_m] -> To Workspace31/1
  Gain32/1 -> To Workspace32/1
  Switch12/1 -> Cut-in strategy/3(TH)
  [Vx_HV_mps] -> Cut-in strategy/4(Vx_HV_mps)
  Cut-in strategy/1(TH*Vx) -> [RR_new], Scope32/1
  [Yaw_HV_deg] -> global to local2/3(Yaw)  "deg"
  [X_HV_m] -> global to local2/1(Xc)
  [Y_HV_m] -> global to local2/2(Yc)
  [X_PV_m] -> global to local2/4(X_ref)
  [Y_PV_m] -> global to local2/5(Y_ref)
  global to local2/1(x_ref) -> [Rx]  "now"
  global to local2/2(y_ref) -> [LeftDis_PV_one], [Ry]  "now"
  Add20/1 -> Mux14/2
  [Rx] -> Add20/1, Mux14/1
  From175/1 -> Add26/1, Scope30/1, Mux15/1
  Add26/1 -> Mux15/2
  Mux15/1 -> Goto95/1, Switch10/1, Scope36/1
  Mux14/1 -> [x_translate]
  Switch10/1 -> descending/1, ascending/1
  From193/1 -> Switch9/2, Switch10/3
  descending/1 -> Switch9/3
  ascending/1 -> Switch9/1
  Switch9/1 -> 11:20/1, 1:10/1
  Manual Switch1/1 -> Goto93/1
  Constant67/1 -> [LaneAvail_flg]
  [LaneAvail_flg] -> R selector/1(In1)
  Demux/12 -> Gain57/1
  Gain57/1 -> Quantizer3/1
  Demux/13 -> Gain59/1
  Gain59/1 -> Quantizer4/1
  Demux/14 -> Gain60/1
  Gain60/1 -> Quantizer5/1
  Demux/15 -> Gain61/1
  Gain61/1 -> Quantizer6/1
  [Roll_rate_L1_radps] -> Add56/1
  [Roll_rate_L2_radps] -> Add56/2
  [Roll_rate_R1_radps] -> Add56/3
  [Roll_rate_R2_radps] -> Add56/4
  Add56/1 -> Gain/1
  Gain/1 -> rolling radius/1
  rolling radius/1 -> Gain56/1
  Gain43/1 -> To Workspace43/1  "est"
  From167/1 -> Gain43/1
  Gain40/1 -> To Workspace42/1  "carsim"
  From166/1 -> Gain40/1
  Constant19/1 -> [OnlyPY_signal]
  Constant38/1 -> Mux17/2
  Gain80/1 -> Vx5/2
  Kalman_Filter_LatSpd1/6(K) -> Display4/1, Scope23/1
  Gain55/1 -> Vx4/3  "small"
  From244/1 -> Gain55/1
  Compare To Constant2/1 -> Switch3/2
  Mux11/1 -> Kalman_Filter_LatSpd1/2(u)
  Kalman_Filter_LatSpd1/4(G) -> Display6/1
  Kalman_Filter_LatSpd1/7(M2) -> Delay48/1
  From257/1 -> Switch3/1
  From241/1 -> Kalman_Filter_LatSpd1/3(Yaw_rate)
  Kalman_Filter_LatSpd1/1(X_e) -> Delay49/1, Demux6/1
  Constant48/1 -> Kalman_Filter_LatSpd1/4(R)
  Constant44/1 -> Kalman_Filter_LatSpd1/5(Q)
  From242/1 -> Switch3/3
  Gain51/1 -> Vx6/1  "carsim"
  From258/1 -> Gain52/1
  Kalman_Filter_LatSpd1/3(F) -> Display5/1
  Demux8/1 -> Gain81/1
  From217/1 -> Scope41/1, Abs6/1
  From255/1 -> Gain54/1
  Gain81/1 -> Vx5/1
  Abs6/1 -> Compare To Constant2/1
  Demux8/2 -> Gain80/1
  Mux17/1 -> Delay49/2
  Demux6/2 -> Goto84/1
  Delay48/1 -> Kalman_Filter_LatSpd1/7(M)
  From247/1 -> Kalman_Filter_LatSpd1/6(y)
  Gain54/1 -> Vx4/2  "Est"
  Kalman_Filter_LatSpd1/2(X_k) -> Demux8/1
  Gain53/1 -> Vx4/1  "carsim"
  Gain52/1 -> Vx6/2  "est1"
  Kalman_Filter_LatSpd1/5(G2) -> Display7/1
  From232/1 -> Gain53/1
  From238/1 -> Gain51/1
  From243/1 -> Mux11/1
  From246/1 -> Mux11/2
  From248/1 -> Mux17/1
  Delay49/1 -> ?
  Demux6/1 -> Goto49/1
  [RR] -> Scope33/1  "RR"
  [RR_new] -> Scope33/2  "RR_new"
  Multiport Switch1/1 -> Cut-in strategy/5(RR)
  [Est_switch] -> Multiport Switch/1
  Constant/1 -> [Est_switch]
  [RR_est] -> Multiport Switch/3
  [Est_switch] -> Multiport Switch1/1
  [RR_est] -> Multiport Switch1/3
  [RR] -> Multiport Switch1/2
  [Est_switch] -> Multiport Switch2/1
  [Est_switch] -> Multiport Switch3/1
  [RR] -> Multiport Switch3/2
  [RR_est] -> Multiport Switch3/3
  [Est_switch] -> Multiport Switch4/1
  [RV_est] -> Multiport Switch4/3
  [RVx] -> Multiport Switch4/2
  cmd_limiter1/1(ax_cmd1) -> Scope34/1, [th_acc]
  Constant58/1 -> Zero-Order Hold3/1
  Constant54/1 -> LateralMotionKF1/8(lr)
  Gain44/1 -> LateralMotionKF1/4(delta)
  Constant56/1 -> LateralMotionKF1/1(T)
  From216/1 -> LateralMotionKF1/2(rk)
  From219/1 -> Unit Delay4/1
  From80/1 -> Display/1, LateralMotionKF1/3(vxk)
  Constant52/1 -> LateralMotionKF1/7(lf)
  Constant57/1 -> LateralMotionKF1/5(Caf)
  Constant59/1 -> LateralMotionKF1/6(Car)
  Constant55/1 -> LateralMotionKF1/9(mv)
  Unit Delay4/1 -> LateralMotionKF1/10(vyk)
  From221/1 -> Gain41/1  "carsim"
  Gain41/1 -> Gain44/1  "deg"
  From233/1 -> Scope50/1
  LateralMotionKF1/1(vyk1) -> Goto90/1, Scope50/2
  1:10/1 -> Manual Switch1/1
  11:20/1 -> Manual Switch1/2
  From234/1 -> Unit Delay5/1
  Unit Delay5/1 -> Mux10/2
  From237/1 -> Delay10/2
  Delay10/1 -> Mux10/1
  From239/1 -> Delay10/1
  Mux10/1 -> Kalman_Filter_LatSpd1/1("X_e ")
  Constant61/1 -> Switch2/3
  Relational Operator3/1 -> Switch2/2
  From253/1 -> Relational Operator3/1
  Constant60/1 -> Relational Operator3/2
  Switch3/1 -> Switch2/1
  Switch2/1 -> Goto91/1
  [Vx_HV_mps] -> R selector/2(vx)
  Multiport Switch5/1 -> [LeftDis_PV]
  Constant62/1 -> Multiport Switch5/1
  [LeftDis_PV_one] -> Multiport Switch5/2
  [LeftDis_PV_multi] -> Multiport Switch5/3
  Mux16/1 -> [yaw_rotate]
  Add62/1 -> Delay50/1, Gain72/1
  T/1 -> Add62/1
  Delay50/1 -> Add62/2
  r/l/1 -> Scope16/2, T/1  "yaw_rate_est"
  Add60/1 -> r/l/1
  [Roll_rate_R1_radps] -> Add60/2
  [Roll_rate_L1_radps] -> Add60/1
  From273/1 -> Reshape/1
  Reshape/1 -> Gain46/1
  [Vx_HV_mps] -> R selector1/2(vx)
  [LaneAvail_flg] -> R selector1/1(In1)
  Gain42/1 -> Cos/1
  Cos/1 -> Product2/2
  Product2/1 -> [delta_y_19]
  [Ry] -> Add32/1, Mux20/1
  Add32/1 -> Mux20/2
  Mux20/1 -> [y_translate]
  [Vx_HV_mps] -> Gain45/1
  record_delta_x/1(delta_x_19) -> [delta_x_19]
  Gain56/1 -> record_delta_x/1(delta_x)
  From188/1 -> Switch10/2
  [delta_x_19] -> Product2/1
  Gain46/1 -> Subsystem6/1(delta__y)
  Subsystem6/1(delta__y_19) -> Add26/2
  Constant63/1 -> Mux16/1
  [delta_yaw] -> Mux16/2
  [delta_yaw] -> Gain42/1
  record_delta_yaw/1(delta_yaw_19) -> Scope56/1, [delta_yaw]
  Gain72/1 -> To Workspace40/1, Scope5/2, record_delta_yaw/1(delta_yaw)  "yaw_est"
  [delta_y_19] -> Add32/2
  [delta_x_19] -> Add20/2
  [Yaw_HV_deg] -> Scope5/1  "carsim"
  [Yaw_rate_radps] -> Scope16/1  "carsim"
  Min/1 -> Scope8/1
  Min1/1 -> [TTC_PV]
  Estimation_TTCx_PV/1(TTC1) -> Scope27/1, Min1/1
  Estimation_TTCx_PV/2(TTC2) -> Scope27/2, Min1/2
  Estimation_TTCx_PV1/2(TTC2) -> Scope43/2, Min2/2
  Estimation_TTCx_PV1/1(TTC1) -> Scope43/1, Min2/1
  Min2/1 -> [TTC_APV]
  [Station_HV_m] -> preview/1(In1)
  [Vx_HV_mps] -> preview/2(In2)
  preview/1(X_ref) -> global to local3/4(X_ref)
  preview/2(Y_ref) -> global to local3/5(Y_ref)
  PV_trajectory_planning/1(LeftDis_PV_multi) -> [LeftDis_PV_multi], Scope58/1
  [x_translate] -> PV_trajectory_planning/1(x_translate)
  [yaw_rotate] -> PV_trajectory_planning/2(yaw_rotate)
  [y_translate] -> PV_trajectory_planning/3(y_translate)
  [Ry] -> PV_trajectory_planning/4(Ry)
  Demux/16 -> Add Constant4/1  "dist_acc"
  Demux/18 -> Gain47/1
  Demux/23 -> [X_PV_m]  "X_Obj_1"
  Demux/17 -> Scope20/1, [VACCTargetVehAssigned_flg]  "DisS1_1"
  Demux/21 -> Gain48/1
  Demux/20 -> [sensor_dectect_y_m]
  Demux/19 -> [sensor_dectect_x_m]
  Demux/24 -> [Y_PV_m]  "Y_Obj_1"
  Add Constant4/1 -> [Desired_distance_carsim_m]
  Gain47/1 -> [sensor_dectect_spd_mps]
  Gain48/1 -> [sensor_dectect_Vx_mps]
  Demux/22 -> Gain49/1
  Gain49/1 -> [sensor_dectect_Vy_mps]
  Demux/25 -> Gain58/1
  Demux/26 -> Gain50/1
  Gain50/1 -> [Ax_PV_mps2]
  Gain58/1 -> [Vx_PV_mps]
  Demux/27 -> [Station_PV_m]
  Demux/32 -> [Station_APV_m]
  Demux/28 -> [X_APV_m]  "X_Obj_3"
  Demux/29 -> [Y_APV_m]  "Y_Obj_3"
  Demux/30 -> Gain1/1
  Gain1/1 -> [Vx_APV_mps]
  Demux/31 -> [Ax_APV_mps2]
  Constant28/1 -> Zero-Order Hold4/1
  [RR_new] -> Mux7/1  "RR"
  [Vx_HV_mps] -> divide2/2(divisor)
  Saturation7/1 -> [TH_plot]  "TH_default"
  divide2/1(quotient) -> Saturation7/1
  Constant7/1 -> divide2/3(default_value)
  Add Constant5/1 -> Abs4/1
  Abs4/1 -> divide2/1(dividend)
  [RR] -> Estimation_TTCx_PV2/1(R)
  [TTC] -> Cut-in strategy/2(TTC)
  [RVx] -> Mux7/2
  Add3/1 -> Scope69/1, divide3/2(divisor), Estimation_TTCx_PV2/2(V)
  Constant20/1 -> divide3/3(default_value)
  Saturation/1 -> Scope68/1, Abs2/1
  [Acc_Mode] -> Switch8/2
  Switch8/1 -> To Workspace11/1
  [Acc_Mode] -> Switch11/2
  [TH_plot] -> Switch11/3  "TH"
  Constant22/1 -> Switch11/1
  V_rel Estimation/1(s_rel) -> [RR_est]
  V_rel Estimation/2(v_rel) -> [RV_est]
  V_rel Estimation/3(a_rel) -> [RA_est]
  [RR] -> Mux4/1
  [Ax_HV_mps2] -> V_rel Estimation/2(a_c)
  [RVx] -> Mux4/2
  [RR] -> V_rel Estimation/3(S_rel)
  [cut_in_flg] -> V_rel Estimation/1(cut_in_flg)
  Mux4/1 -> V_rel Estimation/4(initial_value)
  [RAx] -> Mux4/3
  Subsystem5/4(trig) -> Scope49/1, [cut_in_flg]
  Subsystem5/1(RR) -> Delay9/3, [RR]  "RR"
  [OnlyPY_signal] -> Subsystem5/1(OnlyPV_signal)
  Subsystem7/1(RR_PV) -> Subsystem5/2(RR_PV)
  [RR_APV] -> Subsystem5/5(RR_APV)
  Subsystem7/2(RV_PV) -> Subsystem5/3(RVx_PV)
  [RVx_APV] -> Subsystem5/6(RVx_APV)
  Subsystem7/3(RA_PV) -> Subsystem5/4(RAx_PV)
  [RAx_APV] -> Subsystem5/7(RAx_APV)
  [RY_PV] -> Subsystem5/8(RY_PV)
  [RY_APV] -> Subsystem5/9(RY_APV)
  [RD_PV] -> Subsystem5/10(In10)
  [RD_APV] -> Subsystem5/11(In11)
  Subsystem5/3(RA) -> [RAx]
  [VACCTargetVehAssigned_flg] -> Delay9/2, Subsystem5/Enable
  [VACCTargetVehAssigned_flg] -> Switch12/2
  Gain6/1 -> Scope61/1
  [Vx_PV_mps] -> Gain19/1  "PV"
  Constant8/1 -> Subsystem/1("Trig ")
  [RR] -> Multiport Switch/2
  IC/1 -> [spd_acc]
  [TTC] -> To Workspace29/1
  [Vx_HV_mps] -> Min3/1
  [ACCSetSpeed_mps] -> Min3/2
  Min3/1 -> Add6/2
  [ACCSetSpeed_mps] -> Min4/2
  [Vx_APV_mps] -> Min4/1
  [Vx_HV_mps] -> Add3/2
  [Vx_APV_mps] -> Add3/1
  [RR] -> Scope65/1, divide3/1(dividend)
  Abs2/1 -> Compare To Constant5/1, Detect Increase/1, Scope59/1
  Detect Increase/1 -> Logical Operator3/1
  [TTC_Increase_flg] -> Cut-in strategy/1(TTC_Increase_flg)
  divide3/1(quotient) -> Saturation/1
  Logical Operator3/1 -> Scope66/1, [TTC_Increase_flg]
  Compare To Constant5/1 -> Logical Operator3/2
  [RR] -> Compare To Constant4/1
  Compare To Constant4/1 -> Switch13/2
  Switch13/1 -> [TTC]
  Constant21/1 -> Switch13/1
  Delay1/1 -> Add15/2
  [Yaw_rate_radps] -> Scope70/1  "carsim"
  Add9/1 -> r/l1/1
  Add15/1 -> Delay1/1, Gain5/1
  [Yaw_HV_deg] -> Scope71/1  "carsim"
  [Roll_rate_R1_radps] -> Scope72/2, Quantizer2/1
  [Roll_rate_L1_radps] -> Quantizer1/1
  T1/1 -> Add15/1
  Gain5/1 -> Scope71/2  "yaw_est"
  r/l1/1 -> Scope70/2, T1/1  "yaw_rate_est"
  Quantizer1/1 -> Add9/1
  Quantizer2/1 -> Scope72/1, Add9/2
  Quantizer3/1 -> [Roll_rate_L1_radps]
  Quantizer6/1 -> [Roll_rate_R2_radps]
  Quantizer5/1 -> [Roll_rate_R1_radps]
  Quantizer4/1 -> [Roll_rate_L2_radps]
  Mux/1 -> CarSim S-Function/1
  Subsystem5/2(RV) -> Gain6/1, [RVx]
  Gain11/1 -> Add18/2
  Add18/1 -> Delay9/1, Goto58/1  "RV"
  Delay9/1 -> Add18/1
  [Desired_distance] -> Scope75/1  "Desired_distance"
  [RVx_PV] -> Gain11/1
  [RAx] -> Scope76/1
  [RR] -> Scope75/2
  Divide/1 -> Scope7/1
  [RR] -> Divide/1
  Constant49/1 -> Divide/2
  Subsystem8/1(X_path) -> Camera_NEW/7(X_path)
  Subsystem8/3(s_path) -> Camera_NEW/9(s_path)
  Subsystem8/2(Y_path) -> Camera_NEW/8(Y_path)
  Constant23/1 -> Switch12/3
  [TH] -> Switch12/1
